simulink model "MunozMeneses"  (R2026a)
settings: Solver=ode15s  MaxStep=1e-3
libraries: slpidlib x1, simulink x1
settings Model: Creator=LENOVO
settings DataIOCC: TimeSaveName=t
settings DebuggingCC: ArtificialAlgebraicLoopMsg=none  OperatingPointInterfaceChecksumMismatchMsg=none
settings SimscapeCC: SimscapeNominalValues="[{\"value\":\"1\",\"unit\":\"A\"},{\"value\":\"1\",\"unit\":\"bar\"},{\"value\":\"1\",\"unit\":\"cm^2\"},{\"value\":\"1\",\"unit\":\"cm^3/s\"},{\"value\":\"1\",\"unit\":\"kJ/kg\"},{\"value\":\"1\",\"unit\":\"kW\"},{\"value\":\"1\",\"unit\":\"l\"},{\"value\":\"1\",\"unit\":\"N\"},{\"value\":\"1\",\"unit\":\"N*m\"},{\"value\":\"1\",\"unit\":\"V\"}]"  SimscapeLogType=none  SimscapeLogDataHistory=5000  SimscapeLogDecimation=1

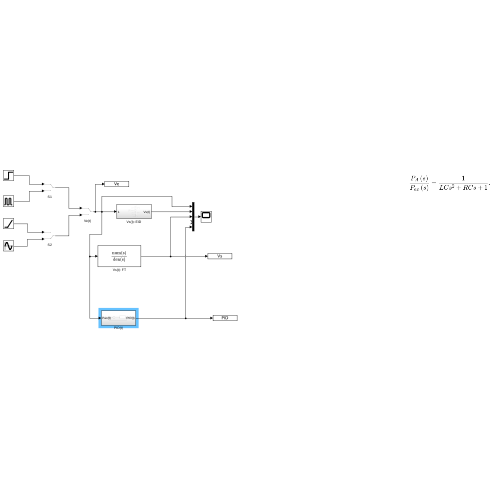
[thumbnail: Simulink's stored preview of the top-level diagram]
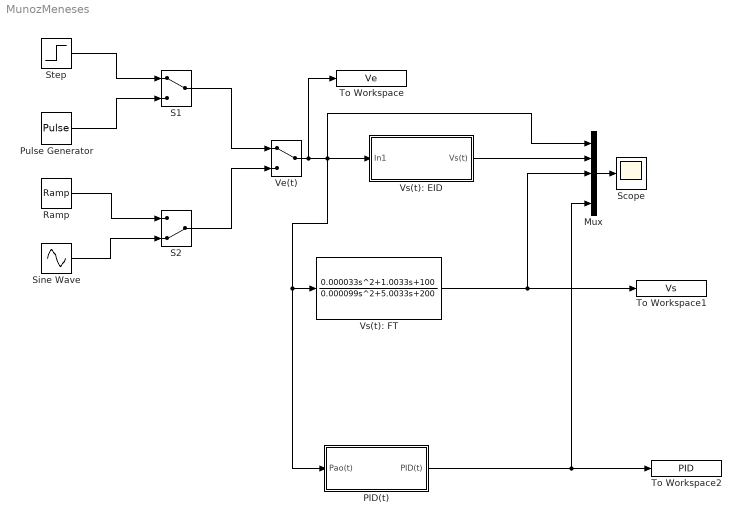
== system MunozMeneses ==
  Mux : Mux  Inputs=5
  PID(t) : Subsystem
  Pulse Generator : DiscretePulseGenerator  PulseType=Time based  Period=10  PulseWidth=10  PhaseDelay=1
  Ramp : simulink/Sources/Ramp  slope=1/10  start=0  InitialOutput=0
  S1 : ManualSwitch
  S2 : ManualSwitch  CurrentSetting=0
  Scope : Scope
      settings: ActiveDisplayYMinimum=-0.16877  ActiveDisplayYMaximum=1.51894
  Sine Wave : Sin  Frequency=pi/2
  Step : Step  Time=0  InitialValue=1  SampleTime=0
  To Workspace : ToWorkspace  VariableName=Ve  SampleTime=-1
  To Workspace1 : ToWorkspace  VariableName=Vs  SampleTime=-1
  To Workspace2 : ToWorkspace  VariableName=PID  SampleTime=-1
  Ve(t) : ManualSwitch
  Vs(t): EID : Subsystem
  Vs(t): FT : TransferFcn  Numerator=[0.000033,1.0033,100]  Denominator=[0.000099,5.0033,200]
  wires:
  Vs(t): EID/1(Vs(t)) -> Mux/2
  Mux/1 -> Scope/1
  Step/1 -> S1/1
  Ve(t)/1 -> To Workspace/1, Mux/1, PID(t)/1(Pao(t)), Vs(t): FT/1, Vs(t): EID/1(In1)
  S1/1 -> Ve(t)/1
  Pulse Generator/1 -> S1/2
  S2/1 -> Ve(t)/2
  Ramp/1 -> S2/1
  Sine Wave/1 -> S2/2
  Vs(t): FT/1 -> Mux/3, To Workspace1/1
  PID(t)/1(PID(t)) -> To Workspace2/1, Mux/5

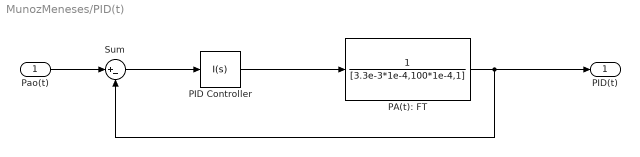
== system MunozMeneses/PID(t) ==
  Pao(t) : Inport
  PA(t): FT : TransferFcn  Denominator=[3.3e-3*1e-4,100*1e-4,1]
  PID Controller : slpidlib/PID Controller  Controller=I  Form=Parallel  TimeDomain=Continuous-time  UseExternalTs=off  SampleTime=-1  IntegratorMethod=Forward Euler  FilterMethod=Forward Euler  ControllerParametersSource=internal  P=1  I=246.4148  UseKiTs=off  D=1  UseExternalDerivativeSource=off  N=1000  UseFilter=on  TunerSelectOption=Transfer Function Based (PID Tuner App)  InitialConditionSource=internal  InitialConditionForIntegrator=0  InitialConditionForFilter=0  DifferentiatorICPrevScaledInput=0  ExternalReset=none  TrackingMode=off  Kt=1  LimitOutput=off  SatLimitsSource=internal  UpperSaturationLimit=inf  LowerSaturationLimit=-inf  LinearizeAsGain=on  AntiWindupMode=none  Kb=1  LimitIntegrator=off  UpperIntegratorSaturationLimit=inf  LowerIntegratorSaturationLimit=-inf  POutMin=[]  POutMax=[]  IOutMin=[]  IOutMax=[]  DOutMin=[]  DOutMax=[]  NOutMin=[]  NOutMax=[]  SumOutMin=[]  SumOutMax=[]  SaturationOutMin=[]  SaturationOutMax=[]  PParamMin=[]  PParamMax=[]  IParamMin=[]  IParamMax=[]  DParamMin=[]  DParamMax=[]  NParamMin=[]  NParamMax=[]  KbParamMin=[]  KbParamMax=[]  KtParamMin=[]  KtParamMax=[]  KbOutMin=[]  KbOutMax=[]  KtOutMin=[]  KtOutMax=[]  IntegratorOutMin=[]  IntegratorOutMax=[]  FilterOutMin=[]  FilterOutMax=[]  SumI1OutMin=[]  SumI1OutMax=[]  SumI2OutMin=[]  SumI2OutMax=[]  SumI3OutMin=[]  SumI3OutMax=[]  SumI4OutMin=[]  SumI4OutMax=[]  SumDOutMin=[]  SumDOutMax=[]  DifferentiatorOutMin=[]  DifferentiatorOutMax=[]  FilterDiffOutCoefMin=[]  FilterDiffOutCoefMax=[]  ReciprocalOutMin=[]  ReciprocalOutMax=[]  SumDenOutMin=[]  SumDenOutMax=[]  SumNumOutMin=[]  SumNumOutMax=[]  DivideOutMin=[]  DivideOutMax=[]  UdiffTsProdOutMin=[]  UdiffTsProdOutMax=[]  NTsProdOutMin=[]  NTsProdOutMax=[]  UintegralTsProdOutMin=[]  UintegralTsProdOutMax=[]  UngainTsProdOutMin=[]  UngainTsProdOutMax=[]  ClampingZeroOutDataTypeStr=Inherit: Inherit via back propagation  ClampingZeroOutMin=[]  ClampingZeroOutMax=[]  FilterDenConstantOutDataTypeStr=Inherit: Inherit via back propagation  FilterDenConstantOutMin=[]  FilterDenConstantOutMax=[]  PCopyOutDataTypeStr=Inherit: Inherit via back propagation  PCopyOutMin=[]  PCopyOutMax=[]  NCopyOutDataTypeStr=Inherit: Inherit via back propagation  NCopyOutMin=[]  NCopyOutMax=[]  IntegratorContinuousStateAttributes=''  IntegratorStateMustResolveToSignalObject=off  IntegratorRTWStateStorageClass=Auto  FilterContinuousStateAttributes=''  FilterStateMustResolveToSignalObject=off  FilterRTWStateStorageClass=Auto  ParallelPVariant=Disabled  IdealPVariant=Disabled  IVariant=InternalParameters  DVariant=Disabled  IntegratorVariant=Continuous  SatVariant=Disabled  AWVariant=Passthrough  PCopyVariant=Disabled  TRVariant=Disabled  FdbkBlocksVariant=Forward  IdealPFdbkVariant=Disabled  SatFdbkVariant=Disabled  DerivativeFilterVariant=Disabled  NVariant=Disabled  NCopyVariant=Disabled_SignalSpec  FilterICVariant=Disabled  IntegratorICVariant=InternalICs  ExternalResetVariant=Disabled  TRSumVariant=Passthrough  SumFdbkVariant=Disabled  SumVariant=Passthrough_I  TsampFilterVariant=InternalTs  TsampNgainVariant=Passthrough  TsampIntegralVariant=Disabled_SignalSpec  ExternalSaturationOutDataTypeStr=Inherit: Same as second input  DerivativeSourceVariant=Disabled  PreIntVariant=InternalPreInt
  Sum : Sum  Inputs=|+-
  PID(t) : Outport
  wires:
  PA(t): FT/1 -> PID(t)/1, Sum/2
  PID Controller/1 -> PA(t): FT/1
  Sum/1 -> PID Controller/1
  Pao(t)/1 -> Sum/1

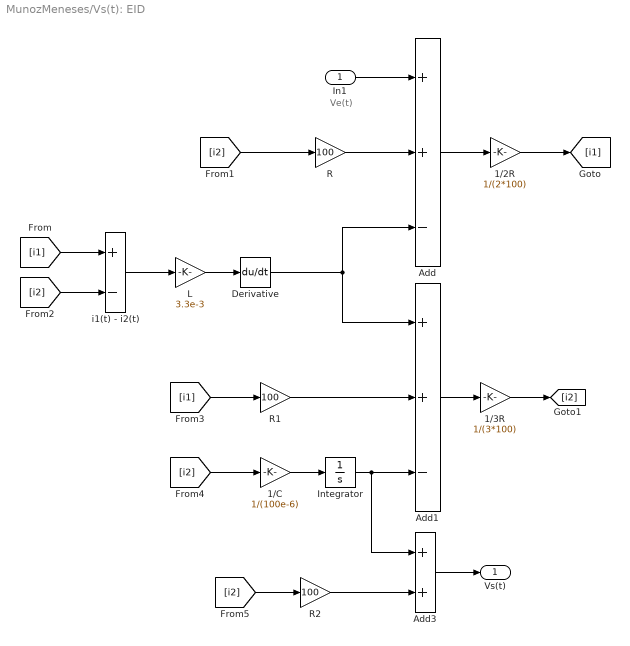
== system MunozMeneses/Vs(t): EID ==
  note: Ve(t)
  In1 : Inport
  1/2R : Gain  Gain=1/(2*100)
  1/3R : Gain  Gain=1/(3*100)
  1/C : Gain  Gain=1/(100e-6)
  Add : Sum  Inputs=++-
  Add1 : Sum  Inputs=++-
  Add3 : Sum
  Derivative : Derivative
  Integrator : Integrator
  L : Gain  Gain=3.3e-3
  R : Gain  Gain=100
  R1 : Gain  Gain=100
  R2 : Gain  Gain=100
  i1(t) - i2(t) : Sum  Inputs=+-
  Vs(t) : Outport
  wires:
  In1/1 -> Add/1
  [i2] -> i1(t) - i2(t)/2
  [i1] -> i1(t) - i2(t)/1
  i1(t) - i2(t)/1 -> L/1
  L/1 -> Derivative/1
  Derivative/1 -> Add/3, Add1/1
  [i1] -> R1/1
  R1/1 -> Add1/2
  Add1/1 -> 1/3R/1
  1/3R/1 -> [i2]
  [i2] -> R/1
  R/1 -> Add/2
  Add/1 -> 1/2R/1
  1/2R/1 -> [i1]
  [i2] -> 1/C/1
  1/C/1 -> Integrator/1
  Integrator/1 -> Add3/1, Add1/3
  [i2] -> R2/1
  R2/1 -> Add3/2
  Add3/1 -> Vs(t)/1
